simulink model "Modelo_no_lineal_completoVA"  (R2017b)
settings: Solver=ode45  StartTime=0.0  StopTime=5  MaxStep=1e-3  RelTol=1e-5  AbsTol=1e-4
values from neighbouring files (symbols this model uses):
  alfacu = 3.9e-3    (= 0.0039)    [datos_motor.m]
  Bl = 0.0530*0    (= 0)    [datos_motor.m]
  Bm = 1.5e-5    (= 1.5e-05)    [datos_motor.m]
  Cts = 1.091    [datos_motor.m]
  f = 60    [datos_motor.m]
  idr0 = 0    [datos_motor.m]
  ioso = 0    [datos_motor.m]
  iqr0 = 0    [datos_motor.m]
  Jl = 0.2520    (= 0.252)    [datos_motor.m]
  Jm = 3.1e-6    (= 3.1e-06)    [datos_motor.m]
  Lamdam = 0.01546    [datos_motor.m]
  Ld = 6.6e-3    (= 0.0066)    [datos_motor.m]
  Lls = 0.8e-3    (= 0.0008)    [datos_motor.m]
  Lq = 5.8e-3    (= 0.0058)    [datos_motor.m]
  Pp = 3    [datos_motor.m]
  r = 314.3008    [datos_motor.m]
  rs = 1.02    [datos_motor.m]
  Rsref = 1.02    [datos_motor.m]
  Rst_amb = 55    [datos_motor.m]
  Tamb = 25    [datos_motor.m]
  theta0 = 0    [datos_motor.m]
  Tref = 40    [datos_motor.m]
  Ts0 = 25    [datos_motor.m]
  vf_a = (24/sqrt(3))*sqrt(2)    [datos_motor.m]
  w0 = 0    [datos_motor.m]
libraries: simulink x3
settings Model: Creator=tomas  LastModifiedBy=Franco
settings CodeAppCC: StateflowObjectComments=on
settings SimscapeCC: SimscapeNormalizeSystem=off

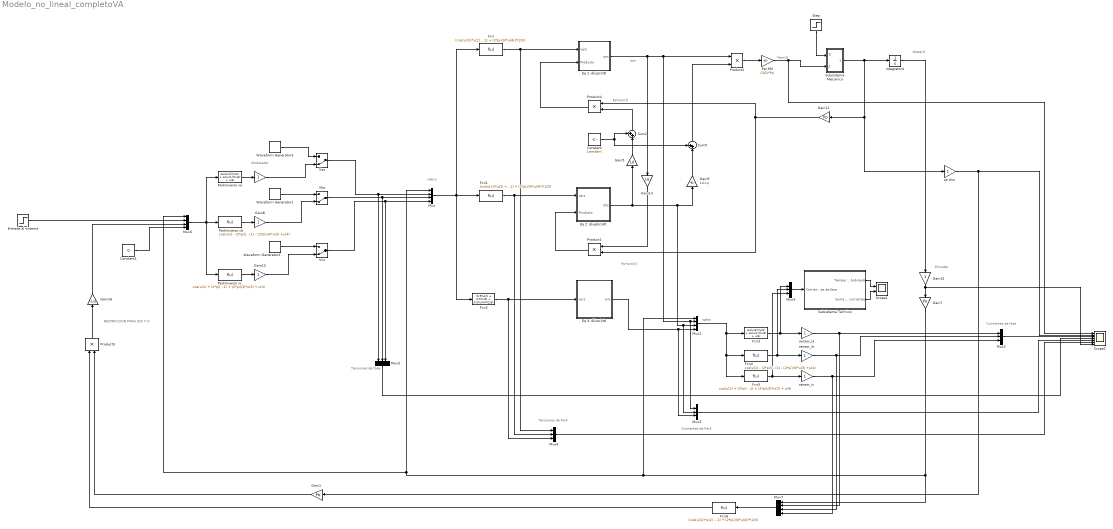
== system Modelo_no_lineal_completoVA ==
  note: Tensiones de Park
  note: Corrientes de Park
  note: Corrientes de fase
  note: Tensiones de fase
  note: vabcs
  note: iqdos
  note: RESTRICCION PARA IDS = 0
  note: Modulador
  note: Encoder
  note: theta(t)
  note: Tem(t)
  note: Pp*wm(t)
  note: Pp*wm(t)
  note: iqrs
  " " : Gain
  "     Eq 1: d(iqsr)/dt" : Subsystem
  Constant : Constant  Value=Lamdam
  Constant1 : Constant  Value=0
  Entrada al sistema : Step  Time=0.1  After=19.596  SampleTime=0
  Eq 2: d(iqdsr)/dt : Subsystem
  Eq 3: d(iosr)/dt : Subsystem
  Fcn : Fcn  Expr=(cos(u(1))*u(2) + cos(u(1) - (2*pi)/3 )*u(3) + cos(u(1) + (2*pi)/3)*u(4))*(2/3)
  Fcn1 : Fcn  Expr=(sin(u(1))*u(2) + sin(u(1) - (2*pi)/3 )*u(3) + sin(u(1) + (2*pi)/3)*u(4))*(2/3)
  Fcn2 : Fcn  Expr=(0.5*u(2) + 0.5*u(3) + 0.5*u(4))*(2/3)
  Fcn3 : Fcn  Expr=cos(u(1))*u(2) + sin(u(1))*u(3) + u(4)
  Fcn4 : Fcn  Expr=cos(u(1) - (2*pi)/3 )*u(2) + sin(u(1) - (2*pi)/3)*u(3) +u(4)
  Fcn5 : Fcn  Expr=cos(u(1) + (2*pi)/3 )*u(2) + sin(u(1) + (2*pi)/3)*u(3) + u(4)
  Fcn6 : Fcn  Expr=(cos(u(1))*u(2) + cos(u(1) - (2*pi)/3 )*u(3) + cos(u(1) + (2*pi)/3)*u(4))*(2/3)
  Gain1 : Gain  Gain=Pp
  Gain11 : Gain  Gain=Pp
  Gain13 : Gain
  Gain14 : Gain  Gain=Lq
  Gain15 : Gain
  Gain16 : Gain  Gain=-Lq
  Gain5 : Gain  Gain=Ld
  Gain7 : Gain  Gain=Pp
  Gain8 : Gain
  Gain9 : Gain  Gain=Ld-Lq
  Integrator4 : Integrator  InitialCondition=theta0
  Mux{,1,6..7} (4 alike) : Mux
  Mux{2..5,9} (5 alike) : Mux  Inputs=3
  Par EM : Gain  Gain=(3/2)*Pp
  ParkInverso va : Fcn  Expr=cos(u(1))*u(2) + sin(u(1))*u(3) + u(4)
  ParkInverso vb : Fcn  Expr=cos(u(1) - (2*pi)/3 )*u(2) + sin(u(1) - (2*pi)/3)*u(3) +u(4)
  ParkInverso vc : Fcn  Expr=cos(u(1) + (2*pi)/3 )*u(2) + sin(u(1) + (2*pi)/3)*u(3) + u(4)
  Product{1..4} (4 alike) : Product
  Scope1 : Scope  NumInputPorts=2
  Scope2 : Scope  NumInputPorts=7
  Step : Step  Time=0.3  After=1.57  SampleTime=0
  Subsistema Mecanico : Subsystem
  Subsistema Termico : Subsystem
  Sum2 : Sum  Inputs=++|
  Sum5 : Sum  Inputs=++|
  Vas : ManualSwitch  CurrentSetting=0
  Vbs : ManualSwitch  CurrentSetting=0
  Vcs : ManualSwitch  CurrentSetting=0
  Waveform Generator1 : simulink/Sources/Waveform Generator  OutMin=[]  OutMax=[]  OutDataTypeStr=double  SelectedSignal=1  Signals=sin(vf_a,f*2*pi,-120*pi/180)#  BlockNames=MultiportSwitch_f5be4ae7152e475#MultiportSwitch_365199b2ec84464  SampleTime=1e-5
      settings: SourceProductName=Simulink
  Waveform Generator2 : simulink/Sources/Waveform Generator  OutMin=[]  OutMax=[]  OutDataTypeStr=double  SelectedSignal=1  Signals=sin(vf_a,f*2*pi,120*pi/180)  BlockNames=MultiportSwitch_cfeb7fdcf937456  SampleTime=1e-5
      settings: SourceProductName=Simulink
  Waveform Generator3 : simulink/Sources/Waveform Generator  OutMin=[]  OutMax=[]  OutDataTypeStr=double  SelectedSignal=1  Signals=sin(vf_a,f*2*pi,0)#  BlockNames=MultiportSwitch_370d4fff2ef74e9#MultiportSwitch_79fa23ace37e4f2  SampleTime=1e-5
      settings: SourceProductName=Simulink
  ob Wm : Gain
  sensor_ia : Gain
  sensor_ib : Gain
  sensor_ic : Gain
  wires:
  Constant/1 -> Sum5/1, Sum2/1
  Gain5/1 -> Sum2/2
  Sum2/1 -> Product4/2
  Mux/1 -> Fcn2/1, Fcn1/1, Fcn/1
  Integrator4/1 -> Gain15/1
  Gain9/1 -> Sum5/2
  Sum5/1 -> Product2/2
  Fcn3/1 -> Mux9/1, sensor_ia/1
  Fcn4/1 -> Mux9/2, sensor_ib/1
  Fcn5/1 -> Mux9/3, sensor_ic/1
  Vas/1 -> Mux/2, Mux3/1
  Vbs/1 -> Mux/3, Mux3/2
  Vcs/1 -> Mux3/3, Mux/4
  Fcn/1 -> Mux4/1, "     Eq 1: d(iqsr)/dt"/1(vqrs)
  Fcn1/1 -> Mux4/2, Eq 2: d(iqdsr)/dt/1(vdrs)
  Fcn2/1 -> Mux4/3, Eq 3: d(iosr)/dt/1(vors)
  Mux1/1 -> Fcn5/1, Fcn4/1, Fcn3/1
  Mux2/1 -> Scope2/3
  Mux3/1 -> Scope2/4
  Gain14/1 -> Product1/1
  Subsistema Mecanico/1(Wm) -> Integrator4/1, ob Wm/1, Gain11/1
  Step/1 -> Subsistema Mecanico/1(Tl)
  Product2/1 -> Par EM/1
  Par EM/1 -> Subsistema Mecanico/2(Tm), Scope2/1
  Mux4/1 -> Scope2/6
  Mux5/1 -> Scope2/5
  Mux6/1 -> ParkInverso va/1, ParkInverso vc/1, ParkInverso vb/1
  Waveform Generator3/1 -> Vas/1
  ParkInverso va/1 -> " "/1
  ParkInverso vb/1 -> Gain8/1
  Waveform Generator1/1 -> Vbs/1
  Waveform Generator2/1 -> Vcs/1
  ParkInverso vc/1 -> Gain13/1
  " "/1 -> Vas/2
  Gain8/1 -> Vbs/2
  Gain13/1 -> Vcs/2
  sensor_ia/1 -> Mux7/2, Mux2/1
  sensor_ib/1 -> Mux7/3, Mux2/2
  sensor_ic/1 -> Mux7/4, Mux2/3
  Gain15/1 -> Scope2/7, Gain7/1
  Gain7/1 -> Mux7/1, Mux1/1, Mux6/1, Mux/1
  Constant1/1 -> Mux6/4
  Entrada al sistema/1 -> Mux6/2
  Gain11/1 -> Product1/2, Product4/1
  Product3/1 -> Gain16/1
  Gain16/1 -> Mux6/3
  Subsistema Termico/1(Temperatura bobinado) -> Scope1/1
  Subsistema Termico/2(Suma cuadratica de corrientes) -> Scope1/2
  "     Eq 1: d(iqsr)/dt"/1(iqrs) -> Mux5/1, Mux1/2, Product2/1, Gain14/1
  Product4/1 -> "     Eq 1: d(iqsr)/dt"/2("Producto ")
  Eq 2: d(iqdsr)/dt/1(idrs) -> Gain5/1, Gain9/1, Mux1/3, Mux5/2
  Product1/1 -> Eq 2: d(iqdsr)/dt/2(Producto)
  Eq 3: d(iosr)/dt/1("iors ") -> Mux5/3, Mux1/4
  ob Wm/1 -> Gain1/1, Scope2/2
  Gain1/1 -> Product3/2
  Mux9/1 -> Subsistema Termico/1(Corrientes de fase)
  Mux7/1 -> Fcn6/1
  Fcn6/1 -> Product3/1

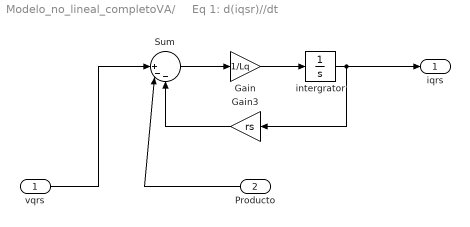
== system Modelo_no_lineal_completoVA/     Eq 1: d(iqsr)//dt ==
  vqrs : Inport
  "Producto " : Inport  Port=2
  Gain : Gain  Gain=1/Lq
  Gain3 : Gain  Gain=rs
  Sum : Sum  Inputs=||+--
  intergrator : Integrator  InitialCondition=iqr0
  iqrs : Outport
  wires:
  vqrs/1 -> Sum/1
  Sum/1 -> Gain/1
  Gain/1 -> intergrator/1
  Gain3/1 -> Sum/3
  "Producto "/1 -> Sum/2
  intergrator/1 -> iqrs/1, Gain3/1

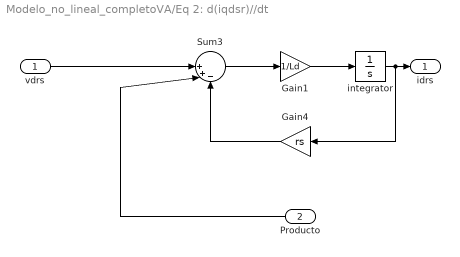
== system Modelo_no_lineal_completoVA/Eq 2: d(iqdsr)//dt ==
  vdrs : Inport
  Producto : Inport  Port=2
  Gain1 : Gain  Gain=1/Ld
  Gain4 : Gain  Gain=rs
  Sum3 : Sum  Inputs=||++-
  integrator : Integrator  InitialCondition=idr0
  idrs : Outport
  wires:
  vdrs/1 -> Sum3/1
  integrator/1 -> Gain4/1, idrs/1
  Gain1/1 -> integrator/1
  Gain4/1 -> Sum3/3
  Producto/1 -> Sum3/2
  Sum3/1 -> Gain1/1

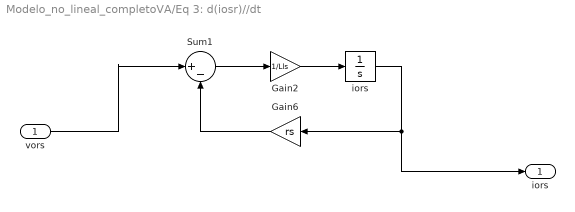
== system Modelo_no_lineal_completoVA/Eq 3: d(iosr)//dt ==
  vors : Inport
  Gain2 : Gain  Gain=1/Lls
  Gain6 : Gain  Gain=rs
  Sum1 : Sum  Inputs=|+-
  iors : Integrator  InitialCondition=ioso
  "iors " : Outport
  wires:
  vors/1 -> Sum1/1
  Gain2/1 -> iors/1
  Sum1/1 -> Gain2/1
  Gain6/1 -> Sum1/2
  iors/1 -> "iors "/1, Gain6/1

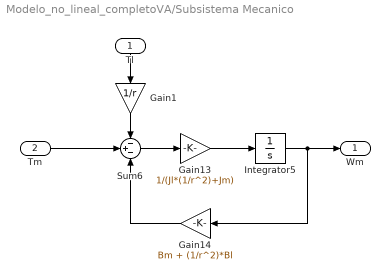
== system Modelo_no_lineal_completoVA/Subsistema Mecanico ==
  Tl : Inport
  Tm : Inport  Port=2
  Gain1 : Gain  Gain=1/r
  Gain13 : Gain  Gain=1/(Jl*(1/r^2)+Jm)
  Gain14 : Gain  Gain=Bm + (1/r^2)*Bl
  Integrator5 : Integrator  InitialCondition=w0
  Sum6 : Sum  Inputs=-+-
  Wm : Outport
  wires:
  Integrator5/1 -> Wm/1, Gain14/1
  Gain14/1 -> Sum6/3
  Tm/1 -> Sum6/2
  Tl/1 -> Gain1/1
  Sum6/1 -> Gain13/1
  Gain13/1 -> Integrator5/1
  Gain1/1 -> Sum6/1

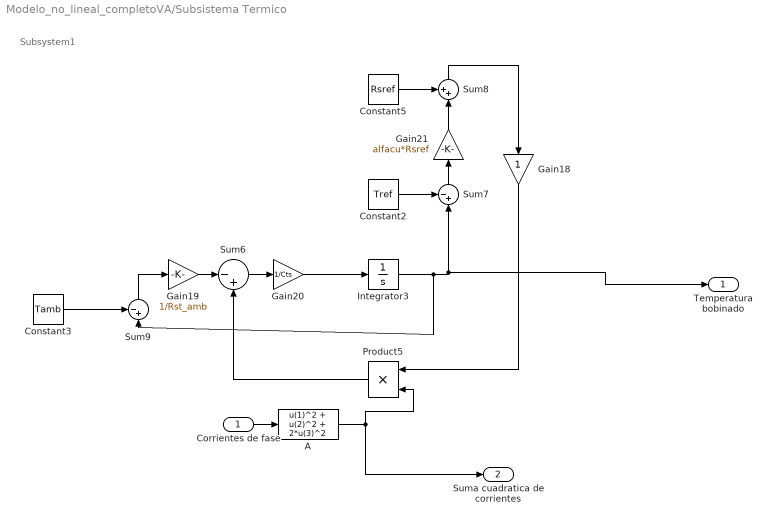
== system Modelo_no_lineal_completoVA/Subsistema Termico ==
  note: Subsystem1
  Corrientes de fase : Inport
  A : Fcn  Expr=u(1)^2 + u(2)^2 + 2*u(3)^2
  Constant2 : Constant  Value=Tref
  Constant3 : Constant  Value=Tamb
  Constant5 : Constant  Value=Rsref
  Gain18 : Gain
  Gain19 : Gain  Gain=1/Rst_amb
  Gain20 : Gain  Gain=1/Cts
  Gain21 : Gain  Gain=alfacu*Rsref
  Integrator3 : Integrator  InitialCondition=Ts0
  Product5 : Product
  Sum6 : Sum  Inputs=|-+
  Sum7 : Sum  Inputs=-+|
  Sum8 : Sum  Inputs=++|
  Sum9 : Sum  Inputs=-+|
  Temperatura bobinado : Outport
  Suma cuadratica de corrientes : Outport  Port=2
  wires:
  Corrientes de fase/1 -> A/1
  Product5/1 -> Sum6/2
  Gain19/1 -> Sum6/1
  Constant2/1 -> Sum7/1
  Gain20/1 -> Integrator3/1
  Integrator3/1 -> Sum9/2, Temperatura bobinado/1, Sum7/2
  Gain18/1 -> Product5/1
  Sum7/1 -> Gain21/1
  Sum8/1 -> Gain18/1
  Sum9/1 -> Gain19/1
  Constant3/1 -> Sum9/1
  Gain21/1 -> Sum8/2
  A/1 -> Suma cuadratica de corrientes/1, Product5/2
  Sum6/1 -> Gain20/1
  Constant5/1 -> Sum8/1
